simulink model "P_I_PI_Controllers"  (R2024b)
settings: Solver=VariableStepAuto  StartTime=0.0  StopTime=100  RelTol=1e-3
settings Model: Creator=LEGION  LastModifiedBy=LEGION

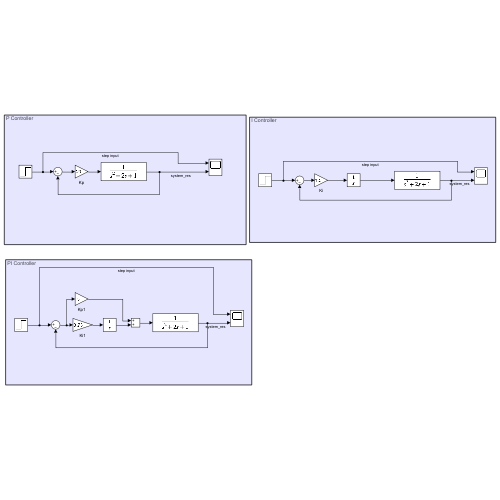
[thumbnail: Simulink's stored preview of the top-level diagram]
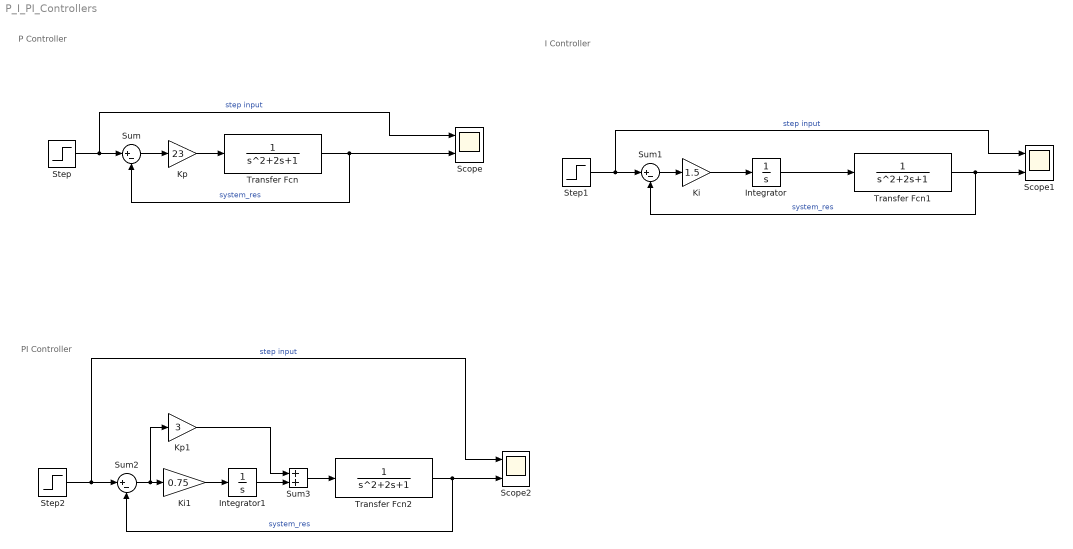
== system P_I_PI_Controllers ==
  note: I Controller
  note: P Controller
  note: PI Controller
  Integrator : Integrator
  Integrator1 : Integrator
  Ki : Gain  Gain=1.5
  Ki1 : Gain  Gain=0.75
  Kp : Gain  Gain=23
  Kp1 : Gain  Gain=3
  Scope : Scope  NumInputPorts=2
  Scope1 : Scope  NumInputPorts=2
  Scope2 : Scope  NumInputPorts=2
  Step : Step  SampleTime=0
  Step1 : Step  SampleTime=0
  Step2 : Step  SampleTime=0
  Sum : Sum  Inputs=|+-
  Sum1 : Sum  Inputs=|+-
  Sum2 : Sum  Inputs=|+-
  Sum3 : Sum
  Transfer Fcn : TransferFcn
  Transfer Fcn1 : TransferFcn
  Transfer Fcn2 : TransferFcn
  wires:
  Step/1 -> Sum/1, Scope/1  "step input"
  Kp/1 -> Transfer Fcn/1
  Transfer Fcn/1 -> Scope/2, Sum/2  "system_res"
  Sum/1 -> Kp/1
  Transfer Fcn1/1 -> Sum1/2, Scope1/2  "system_res"
  Sum1/1 -> Ki/1
  Step1/1 -> Scope1/1, Sum1/1  "step input"
  Integrator/1 -> Transfer Fcn1/1
  Ki/1 -> Integrator/1
  Ki1/1 -> Integrator1/1
  Sum2/1 -> Kp1/1, Ki1/1
  Transfer Fcn2/1 -> Sum2/2, Scope2/2  "system_res"
  Step2/1 -> Scope2/1, Sum2/1  "step input"
  Sum3/1 -> Transfer Fcn2/1
  Integrator1/1 -> Sum3/2
  Kp1/1 -> Sum3/1
